simulink model "bh_4bar_model_DYN"  (R2022b)
settings: Solver=ode45  StartTime=0.0  StopTime=10  FixedStep=0.001  MaxStep=0.1  RelTol=1e-9  AbsTol=1e-9  EnableMultiTasking=on
values from neighbouring files (symbols this model uses):
  L1 = 0.4    [bh_4bar_kin_z_analysis_CLS.m]
  L2 = 1.4    [bh_4bar_kin_z_analysis_CLS.m]
  L3 = 1.2    [bh_4bar_kin_z_analysis_CLS.m]
  L4 = 1    [bh_4bar_kin_z_analysis_CLS.m]
  N = length(THE_DEG_ANG_VEC)    [bh_4bar_kin_z_analysis_CLS.m]
  X = my_stuff_T.theta_deg_vec    [bh_4bar_kin_z_analysis_CLS.m]
undefined symbols (not defined in the file or in its folder): alpha_0_rad, alpha_dot_0_rad, alpha_rad, g, H, I_G1, I_G2, I_G3, m1, m2, m3, phi_0_rad, phi_dot_0_rad, phi_rad, theta_0_rad, theta_dot_0_rad, W, Y, Z
libraries: nesl_utility x20, sm_lib x15, simulink_extras x14, bh_4bar_SL_LIB x13
(part 1 of 3)
settings Model: Creator=bhorton  LastModifiedBy=bhorton
settings SolverCC: ZeroCrossAlgorithm=Adaptive  AlgebraicLoopSolver=TrustRegion
settings DataIOCC: LimitDataPoints=on  ReturnWorkspaceOutputs=off
settings OptimizationCC: LifeSpan=inf
settings DebuggingCC: UnconnectedInputMsg=warning  UnconnectedOutputMsg=warning  UnconnectedLineMsg=warning  AllowSymbolicDim=off  PregeneratedLibrarySubsystemCodeDiagnostic=none  SFUnexpectedBacktrackingDiag=warning  SFNoUnconditionalDefaultTransitionDiag=warning  SFExecutionAtInitializationDiag=none  SFMachineParentedDataDiag=warning  ArithmeticOperatorsInVariantConditions=warning
settings ModelReferenceCC: EnableRefExpFcnMdlSchedulingChecks=on
settings SFSimCC: SimUseLocalCustomCode=off  CustomCodeUndefinedFunction=UseInterfaceOnly
settings RTWCC: RTWUseLocalCustomCode=off  DLArmComputeVersion=19.05
settings CodeAppCC: StateflowObjectComments=on
settings GRTTargetCC: TargetLangStandard=C89/C90 (ANSI)
settings ConfigComp: CovMetricSettings=dw  CovSaveCumulativeToWorkspaceVar=on  CovSaveSingleToWorkspaceVar=on  CovExternalEMLEnable=off  CovSFcnEnable=off
settings SimscapeCC: SimscapeNominalValues="[{\"value\":\"10\",\"unit\":\"V\"},{\"value\":\"1\",\"unit\":\"A\"},{\"value\":\"10\",\"unit\":\"N*m\"},{\"value\":\"10\",\"unit\":\"bar\"},{\"value\":\"100\",\"unit\":\"kJ/kg\"},{\"value\":\"1\",\"unit\":\"kW\"},{\"value\":\"300\",\"unit\":\"K\"},{\"value\":\"100\",\"unit\":\"cm^3/s\"},{\"value\":\"1\",\"unit\":\"kN\"},{\"value\":\"1\",\"unit\":\"g/cm^3\"},{\"value\":\"1\",\"unit\":\"l\"},{\"value\":\"1\",\"unit\":\"cm^2\"},{\"value\":\"60\",\"unit\":\"Hz\"}]"  SimscapeLogType=all  SimscapeLogDataHistory=10000
settings ConfigurationSet: Description=SimMechanics 2G
settings ExplorerConfigSet: InternalSimMechanicsExplorerSettings="<ExplorerConfiguration><canonicalview>default</canonicalview><AnimationSetting><BasePlaybackSpeed>1.0</BasePlaybackSpeed><PlaybackSpeedFactor>1.0</PlaybackSpeedFactor></AnimationSetting><TilePanel><TileInfo><Tiles Columns=\"1\" Count=\"1\" Rows=\"1\"><Column Weight=\"1\"/><Row Weight=\"1\"/><Tile Height=\"1\" Width=\"1\" X=\"0\" Y=\"0\"/></Tiles></TileInfo><SceneInfo><SceneViewer><BGColor><R>0.60000002384185791</R><G>0.60000002384185791</G><B>0.60000002384185791</B></BGColor><Camera><DoPerspective>off</DoPerspective><Position><X>0.674057005362880823</X><Y>0.451513124756151407</Y><Z>1.11774542835223722</Z></Position><Center><X>0.674057005362880823</X><Y>0.451513124756151407</Y><Z>-0.00200006458294343936</Z></Center><Up><X>0</X><Y>1</Y><Z>-0</Z></Up><ViewLimDist>1</ViewLimDist><YLim>0.872355052534568132</YLim><XLim>1.30853257880185225</XLim></Camera></SceneViewer></SceneInfo></TilePanel><MechEditorPanel><Cameras/><GfxPanelCameraMap/><VideoCreator><PlaybackSpeedRatio>1.0</PlaybackSpeedRatio><FrameRate>30</FrameRate><VideoFormat>Motion JPEG AVI</VideoFormat><FrameSize>auto</FrameSize></VideoCreator></MechEditorPanel></ExplorerConfiguration>"

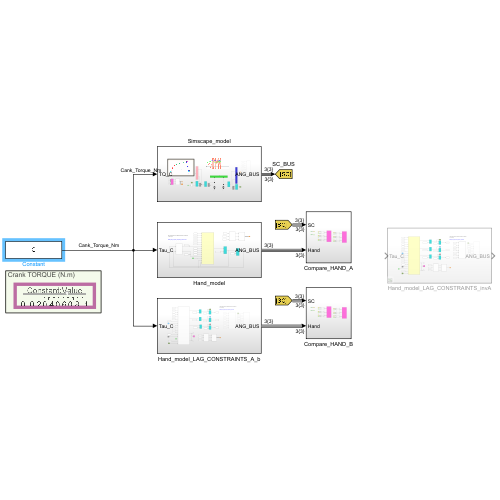
[thumbnail: Simulink's stored preview of the top-level diagram]
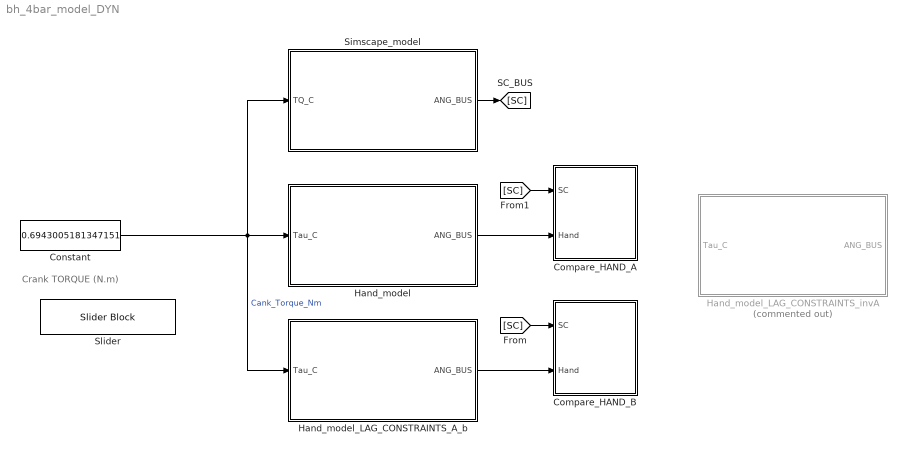
== system bh_4bar_model_DYN ==
  note: Crank TORQUE (N.m)
  Compare_HAND_A : Subsystem
  Compare_HAND_B : Subsystem
  Constant : Constant  Value=0.6943005181347151
  Hand_model : Subsystem
  Hand_model_LAG_CONSTRAINTS_A_b : Subsystem
  Hand_model_LAG_CONSTRAINTS_invA : Subsystem  Commented=on
  Simscape_model : Subsystem
  Slider : SliderBlock  ScaleMax=1
  wires:
  Constant/1 -> Hand_model_LAG_CONSTRAINTS_A_b/1(Tau_C), Simscape_model/1(TQ_C), Hand_model/1(Tau_C)  "Cank_Torque_Nm"
  Simscape_model/1(ANG_BUS) -> [SC]
  Hand_model/1(ANG_BUS) -> Compare_HAND_A/2(Hand)
  Hand_model_LAG_CONSTRAINTS_A_b/1(ANG_BUS) -> Compare_HAND_B/2(Hand)
  [SC] -> Compare_HAND_B/1(SC)
  [SC] -> Compare_HAND_A/1(SC)

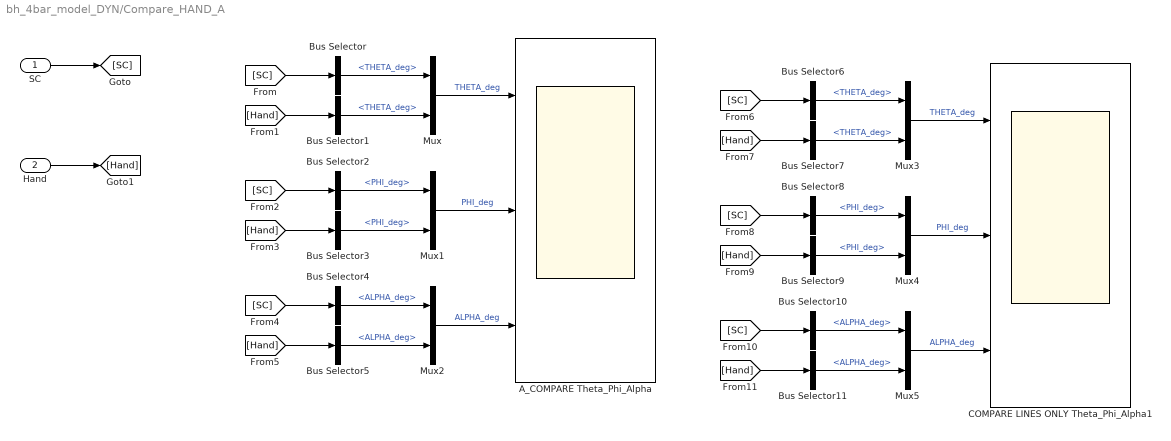
== system bh_4bar_model_DYN/Compare_HAND_A ==
  SC : Inport
  Hand : Inport  Port=2
  A_COMPARE Theta_Phi_Alpha : Scope  NumInputPorts=3
  Bus Selector{,1,6..7} (4 alike) : BusSelector  OutputSignals=THETA_deg
  Bus Selector{4..5,10..11} (4 alike) : BusSelector  OutputSignals=ALPHA_deg
  Bus Selector{2..3,8..9} (4 alike) : BusSelector  OutputSignals=PHI_deg
  COMPARE LINES ONLY Theta_Phi_Alpha1 : Scope  NumInputPorts=3
  Mux{,1..5} (6 alike) : Mux  Inputs=2
  wires:
  Hand/1 -> [Hand]
  SC/1 -> [SC]
  Mux/1 -> A_COMPARE Theta_Phi_Alpha/1  "THETA_deg"
  [SC] -> Bus Selector/1
  Bus Selector/1 -> Mux/1  "<THETA_deg>"
  [Hand] -> Bus Selector1/1
  Bus Selector1/1 -> Mux/2  "<THETA_deg>"
  Mux1/1 -> A_COMPARE Theta_Phi_Alpha/2  "PHI_deg"
  [SC] -> Bus Selector2/1
  Bus Selector3/1 -> Mux1/2  "<PHI_deg>"
  [Hand] -> Bus Selector3/1
  Bus Selector2/1 -> Mux1/1  "<PHI_deg>"
  Mux2/1 -> A_COMPARE Theta_Phi_Alpha/3  "ALPHA_deg"
  [Hand] -> Bus Selector5/1
  [SC] -> Bus Selector4/1
  Bus Selector5/1 -> Mux2/2  "<ALPHA_deg>"
  Bus Selector4/1 -> Mux2/1  "<ALPHA_deg>"
  Bus Selector10/1 -> Mux5/1  "<ALPHA_deg>"
  [Hand] -> Bus Selector11/1
  Mux5/1 -> COMPARE LINES ONLY Theta_Phi_Alpha1/3  "ALPHA_deg"
  Bus Selector11/1 -> Mux5/2  "<ALPHA_deg>"
  Mux4/1 -> COMPARE LINES ONLY Theta_Phi_Alpha1/2  "PHI_deg"
  [Hand] -> Bus Selector7/1
  Bus Selector8/1 -> Mux4/1  "<PHI_deg>"
  [SC] -> Bus Selector6/1
  Mux3/1 -> COMPARE LINES ONLY Theta_Phi_Alpha1/1  "THETA_deg"
  Bus Selector6/1 -> Mux3/1  "<THETA_deg>"
  [Hand] -> Bus Selector9/1
  [SC] -> Bus Selector8/1
  Bus Selector7/1 -> Mux3/2  "<THETA_deg>"
  [SC] -> Bus Selector10/1
  Bus Selector9/1 -> Mux4/2  "<PHI_deg>"

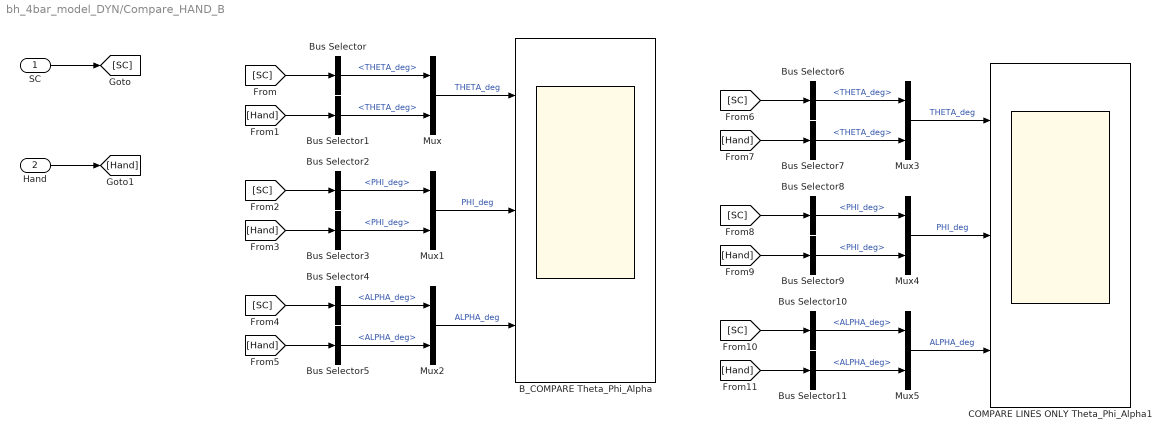
== system bh_4bar_model_DYN/Compare_HAND_B ==
  SC : Inport
  Hand : Inport  Port=2
  B_COMPARE Theta_Phi_Alpha : Scope  NumInputPorts=3
  Bus Selector{,1,6..7} (4 alike) : BusSelector  OutputSignals=THETA_deg
  Bus Selector{4..5,10..11} (4 alike) : BusSelector  OutputSignals=ALPHA_deg
  Bus Selector{2..3,8..9} (4 alike) : BusSelector  OutputSignals=PHI_deg
  COMPARE LINES ONLY Theta_Phi_Alpha1 : Scope  NumInputPorts=3
  Mux{,1..5} (6 alike) : Mux  Inputs=2
  wires:
  Hand/1 -> [Hand]
  SC/1 -> [SC]
  Mux/1 -> B_COMPARE Theta_Phi_Alpha/1  "THETA_deg"
  [SC] -> Bus Selector/1
  Bus Selector/1 -> Mux/1  "<THETA_deg>"
  [Hand] -> Bus Selector1/1
  Bus Selector1/1 -> Mux/2  "<THETA_deg>"
  Mux1/1 -> B_COMPARE Theta_Phi_Alpha/2  "PHI_deg"
  [SC] -> Bus Selector2/1
  Bus Selector3/1 -> Mux1/2  "<PHI_deg>"
  [Hand] -> Bus Selector3/1
  Bus Selector2/1 -> Mux1/1  "<PHI_deg>"
  Mux2/1 -> B_COMPARE Theta_Phi_Alpha/3  "ALPHA_deg"
  [Hand] -> Bus Selector5/1
  [SC] -> Bus Selector4/1
  Bus Selector5/1 -> Mux2/2  "<ALPHA_deg>"
  Bus Selector4/1 -> Mux2/1  "<ALPHA_deg>"
  Bus Selector10/1 -> Mux5/1  "<ALPHA_deg>"
  [Hand] -> Bus Selector11/1
  Mux5/1 -> COMPARE LINES ONLY Theta_Phi_Alpha1/3  "ALPHA_deg"
  Bus Selector11/1 -> Mux5/2  "<ALPHA_deg>"
  Mux4/1 -> COMPARE LINES ONLY Theta_Phi_Alpha1/2  "PHI_deg"
  [Hand] -> Bus Selector7/1
  Bus Selector8/1 -> Mux4/1  "<PHI_deg>"
  [SC] -> Bus Selector6/1
  Mux3/1 -> COMPARE LINES ONLY Theta_Phi_Alpha1/1  "THETA_deg"
  Bus Selector6/1 -> Mux3/1  "<THETA_deg>"
  [Hand] -> Bus Selector9/1
  [SC] -> Bus Selector8/1
  Bus Selector7/1 -> Mux3/2  "<THETA_deg>"
  [SC] -> Bus Selector10/1
  Bus Selector9/1 -> Mux4/2  "<PHI_deg>"

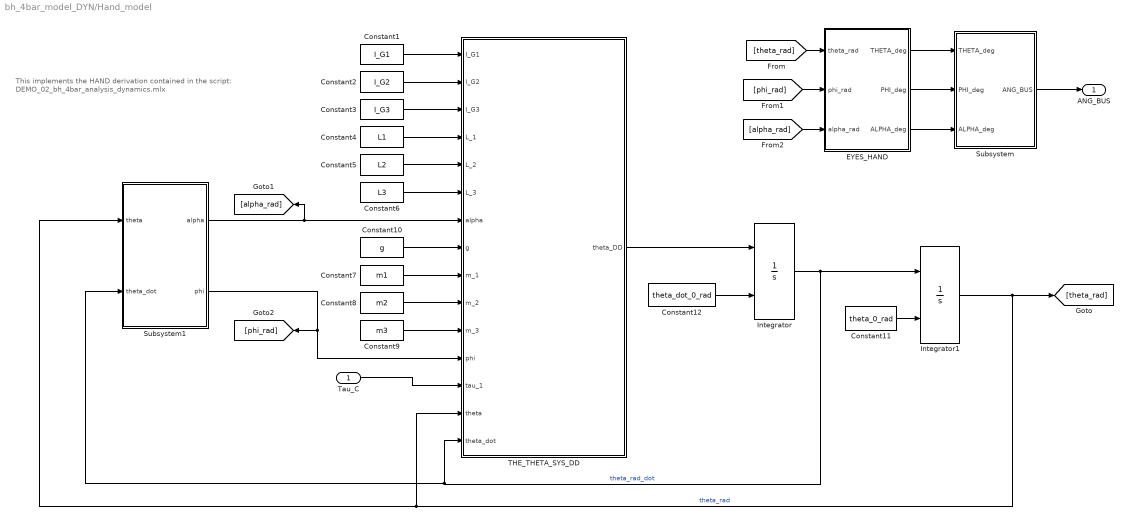
== system bh_4bar_model_DYN/Hand_model ==
  note: This implements the HAND derivation contained
      | in the script:
      |
      | DEMO_02_bh_4bar_analysis_dynamics.mlx
  Tau_C : Inport
  Constant1 : Constant  Value=I_G1
  Constant10 : Constant  Value=g
  Constant11 : Constant  Value=theta_0_rad
  Constant12 : Constant  Value=theta_dot_0_rad
  Constant2 : Constant  Value=I_G2
  Constant3 : Constant  Value=I_G3
  Constant4 : Constant  Value=L1
  Constant5 : Constant  Value=L2
  Constant6 : Constant  Value=L3
  Constant7 : Constant  Value=m1
  Constant8 : Constant  Value=m2
  Constant9 : Constant  Value=m3
  EYES_HAND : Subsystem
  Integrator : Integrator  InitialConditionSource=external
  Integrator1 : Integrator  InitialConditionSource=external
  Subsystem : Subsystem
  Subsystem1 : Subsystem
  THE_THETA_SYS_DD : MATLAB Function  TreatAsAtomicUnit=on
  ANG_BUS : Outport  VectorParamsAs1DForOutWhenUnconnected=off
  wires:
  Constant7/1 -> THE_THETA_SYS_DD/9(m_1)
  Constant8/1 -> THE_THETA_SYS_DD/10(m_2)
  Integrator/1 -> THE_THETA_SYS_DD/15(theta_dot), Subsystem1/2(theta_dot), Integrator1/1  "theta_rad_dot"
  Subsystem1/1(alpha) -> THE_THETA_SYS_DD/7(alpha), [alpha_rad]
  Constant6/1 -> THE_THETA_SYS_DD/6(L_3)
  Integrator1/1 -> [theta_rad], THE_THETA_SYS_DD/14(theta), Subsystem1/1(theta)  "theta_rad"
  Subsystem/1(ANG_BUS) -> ANG_BUS/1
  Constant5/1 -> THE_THETA_SYS_DD/5(L_2)
  EYES_HAND/2(PHI_deg) -> Subsystem/2(PHI_deg)
  EYES_HAND/1(THETA_deg) -> Subsystem/1(THETA_deg)
  EYES_HAND/3(ALPHA_deg) -> Subsystem/3(ALPHA_deg)
  Subsystem1/2(phi) -> THE_THETA_SYS_DD/12(phi), [phi_rad]
  [theta_rad] -> EYES_HAND/1(theta_rad)
  [phi_rad] -> EYES_HAND/2(phi_rad)
  THE_THETA_SYS_DD/1(theta_DD) -> Integrator/1
  [alpha_rad] -> EYES_HAND/3(alpha_rad)
  Constant3/1 -> THE_THETA_SYS_DD/3(I_G3)
  Constant2/1 -> THE_THETA_SYS_DD/2(I_G2)
  Constant4/1 -> THE_THETA_SYS_DD/4(L_1)
  Constant10/1 -> THE_THETA_SYS_DD/8(g)
  Constant9/1 -> THE_THETA_SYS_DD/11(m_3)
  Constant1/1 -> THE_THETA_SYS_DD/1(I_G1)
  Tau_C/1 -> THE_THETA_SYS_DD/13(tau_1)
  Constant12/1 -> Integrator/2
  Constant11/1 -> Integrator1/2

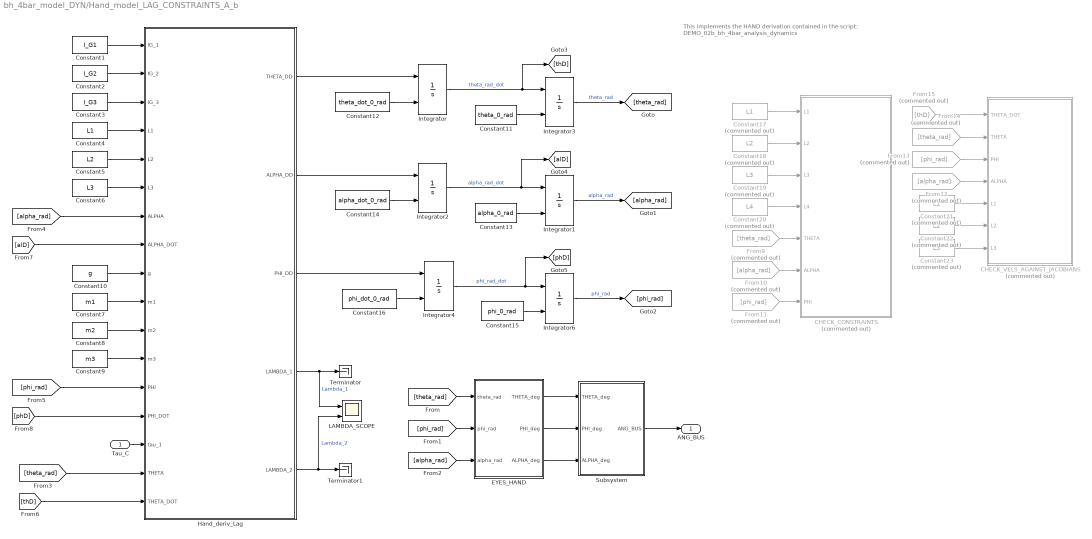
== system bh_4bar_model_DYN/Hand_model_LAG_CONSTRAINTS_A_b ==
  note: This implements the HAND derivation contained
      | in the script:
      |
      | DEMO_02b_bh_4bar_analysis_dynamics
  Tau_C : Inport
  CHECK_CONSTRAINTS : Subsystem  Commented=on
  CHECK_VELS_AGAINST_JACOBIANS : Subsystem  Commented=on
  Constant1 : Constant  Value=I_G1
  Constant10 : Constant  Value=g
  Constant11 : Constant  Value=theta_0_rad
  Constant12 : Constant  Value=theta_dot_0_rad
  Constant13 : Constant  Value=alpha_0_rad
  Constant14 : Constant  Value=alpha_dot_0_rad
  Constant15 : Constant  Value=phi_0_rad
  Constant16 : Constant  Value=phi_dot_0_rad
  Constant17 : Constant  Commented=on  Value=L1
  Constant18 : Constant  Commented=on  Value=L2
  Constant19 : Constant  Commented=on  Value=L3
  Constant2 : Constant  Value=I_G2
  Constant20 : Constant  Commented=on  Value=L4
  Constant21 : Constant  Commented=on  Value=L1
  Constant22 : Constant  Commented=on  Value=L2
  Constant23 : Constant  Commented=on  Value=L3
  Constant3 : Constant  Value=I_G3
  Constant4 : Constant  Value=L1
  Constant5 : Constant  Value=L2
  Constant6 : Constant  Value=L3
  Constant7 : Constant  Value=m1
  Constant8 : Constant  Value=m2
  Constant9 : Constant  Value=m3
  EYES_HAND : Subsystem
  From10 : From  Commented=on  GotoTag=alpha_rad
  From11 : From  Commented=on  GotoTag=phi_rad
  From12 : From  Commented=on  GotoTag=alpha_rad
  From13 : From  Commented=on  GotoTag=phi_rad
  From14 : From  Commented=on  GotoTag=theta_rad
  From15 : From  Commented=on  GotoTag=thD
  From9 : From  Commented=on  GotoTag=theta_rad
  Hand_deriv_Lag : Subsystem
  Integrator : Integrator  InitialConditionSource=external
  Integrator1 : Integrator  InitialConditionSource=external  WrapState=on
  Integrator2 : Integrator  InitialConditionSource=external
  Integrator3 : Integrator  InitialConditionSource=external  WrapState=on
  Integrator4 : Integrator  InitialConditionSource=external
  Integrator6 : Integrator  InitialConditionSource=external  WrapState=on
  LAMBDA_SCOPE : Scope  NumInputPorts=2
  Subsystem : Subsystem
  Terminator : Terminator
  Terminator1 : Terminator
  ANG_BUS : Outport  VectorParamsAs1DForOutWhenUnconnected=off
  wires:
  Constant7/1 -> Hand_deriv_Lag/10(m1)
  Constant8/1 -> Hand_deriv_Lag/11(m2)
  Integrator/1 -> Integrator3/1, [thD]  "theta_rad_dot"
  Constant6/1 -> Hand_deriv_Lag/6(L3)
  Integrator3/1 -> [theta_rad]  "theta_rad"
  Subsystem/1(ANG_BUS) -> ANG_BUS/1
  Constant5/1 -> Hand_deriv_Lag/5(L2)
  EYES_HAND/2(PHI_deg) -> Subsystem/2(PHI_deg)
  EYES_HAND/1(THETA_deg) -> Subsystem/1(THETA_deg)
  EYES_HAND/3(ALPHA_deg) -> Subsystem/3(ALPHA_deg)
  [theta_rad] -> EYES_HAND/1(theta_rad)
  [phi_rad] -> EYES_HAND/2(phi_rad)
  Hand_deriv_Lag/1(THETA_DD) -> Integrator/1
  [alpha_rad] -> EYES_HAND/3(alpha_rad)
  Constant3/1 -> Hand_deriv_Lag/3(IG_3)
  Constant2/1 -> Hand_deriv_Lag/2(IG_2)
  Constant4/1 -> Hand_deriv_Lag/4(L1)
  Constant10/1 -> Hand_deriv_Lag/9(g)
  Constant9/1 -> Hand_deriv_Lag/12(m3)
  Constant1/1 -> Hand_deriv_Lag/1(IG_1)
  Tau_C/1 -> Hand_deriv_Lag/15(tau_1)
  Constant12/1 -> Integrator/2
  Constant11/1 -> Integrator3/2
  Integrator2/1 -> Integrator1/1, [alD]  "alpha_rad_dot"
  Hand_deriv_Lag/2(ALPHA_DD) -> Integrator2/1
  Constant13/1 -> Integrator1/2
  Integrator1/1 -> [alpha_rad]  "alpha_rad"
  Constant14/1 -> Integrator2/2
  Constant15/1 -> Integrator6/2
  Integrator4/1 -> Integrator6/1, [phD]  "phi_rad_dot"
  Integrator6/1 -> [phi_rad]  "phi_rad"
  Constant16/1 -> Integrator4/2
  Hand_deriv_Lag/3(PHI_DD) -> Integrator4/1
  Hand_deriv_Lag/4(LAMBDA_1) -> LAMBDA_SCOPE/1, Terminator/1  "Lambda_1"
  Hand_deriv_Lag/5(LAMBDA_2) -> LAMBDA_SCOPE/2, Terminator1/1  "Lambda_2"
  [theta_rad] -> Hand_deriv_Lag/16(THETA)
  [thD] -> Hand_deriv_Lag/17(THETA_DOT)
  [phD] -> Hand_deriv_Lag/14(PHI_DOT)
  [phi_rad] -> Hand_deriv_Lag/13(PHI)
  [alD] -> Hand_deriv_Lag/8(ALPHA_DOT)
  [alpha_rad] -> Hand_deriv_Lag/7(ALPHA)
  Constant17/1 -> CHECK_CONSTRAINTS/1(L1)
  Constant18/1 -> CHECK_CONSTRAINTS/2(L2)
  Constant19/1 -> CHECK_CONSTRAINTS/3(L3)
  Constant20/1 -> CHECK_CONSTRAINTS/4(L4)
  From9/1 -> CHECK_CONSTRAINTS/5(THETA)
  From10/1 -> CHECK_CONSTRAINTS/6(ALPHA)
  From11/1 -> CHECK_CONSTRAINTS/7(PHI)
  From15/1 -> CHECK_VELS_AGAINST_JACOBIANS/1(THETA_DOT)
  From14/1 -> CHECK_VELS_AGAINST_JACOBIANS/2(THETA)
  From13/1 -> CHECK_VELS_AGAINST_JACOBIANS/3(PHI)
  From12/1 -> CHECK_VELS_AGAINST_JACOBIANS/4(ALPHA)
  Constant21/1 -> CHECK_VELS_AGAINST_JACOBIANS/5(L1)
  Constant22/1 -> CHECK_VELS_AGAINST_JACOBIANS/6(L2)
  Constant23/1 -> CHECK_VELS_AGAINST_JACOBIANS/7(L3)

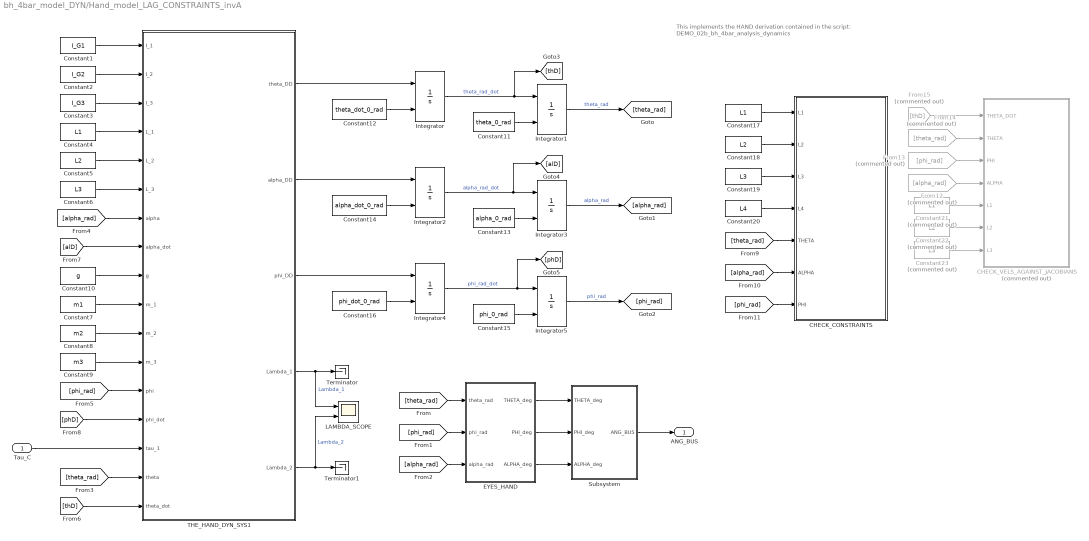
== system bh_4bar_model_DYN/Hand_model_LAG_CONSTRAINTS_invA ==
  note: This implements the HAND derivation contained
      | in the script:
      |
      | DEMO_02b_bh_4bar_analysis_dynamics
  Tau_C : Inport
  CHECK_CONSTRAINTS : Subsystem
  CHECK_VELS_AGAINST_JACOBIANS : Subsystem  Commented=on
  Constant1 : Constant  Value=I_G1
  Constant10 : Constant  Value=g
  Constant11 : Constant  Value=theta_0_rad
  Constant12 : Constant  Value=theta_dot_0_rad
  Constant13 : Constant  Value=alpha_0_rad
  Constant14 : Constant  Value=alpha_dot_0_rad
  Constant15 : Constant  Value=phi_0_rad
  Constant16 : Constant  Value=phi_dot_0_rad
  Constant17 : Constant  Value=L1
  Constant18 : Constant  Value=L2
  Constant19 : Constant  Value=L3
  Constant2 : Constant  Value=I_G2
  Constant20 : Constant  Value=L4
  Constant21 : Constant  Commented=on  Value=L1
  Constant22 : Constant  Commented=on  Value=L2
  Constant23 : Constant  Commented=on  Value=L3
  Constant3 : Constant  Value=I_G3
  Constant4 : Constant  Value=L1
  Constant5 : Constant  Value=L2
  Constant6 : Constant  Value=L3
  Constant7 : Constant  Value=m1
  Constant8 : Constant  Value=m2
  Constant9 : Constant  Value=m3
  EYES_HAND : Subsystem
  From12 : From  Commented=on  GotoTag=alpha_rad
  From13 : From  Commented=on  GotoTag=phi_rad
  From14 : From  Commented=on  GotoTag=theta_rad
  From15 : From  Commented=on  GotoTag=thD
  Integrator : Integrator  InitialConditionSource=external
  Integrator1 : Integrator  InitialConditionSource=external  WrapState=on
  Integrator2 : Integrator  InitialConditionSource=external
  Integrator3 : Integrator  InitialConditionSource=external  WrapState=on
  Integrator4 : Integrator  InitialConditionSource=external
  Integrator5 : Integrator  InitialConditionSource=external  WrapState=on
  LAMBDA_SCOPE : Scope  NumInputPorts=2
  Subsystem : Subsystem
  THE_HAND_DYN_SYS1 : MATLAB Function  TreatAsAtomicUnit=on
  Terminator : Terminator
  Terminator1 : Terminator
  ANG_BUS : Outport  VectorParamsAs1DForOutWhenUnconnected=off
  wires:
  Constant7/1 -> THE_HAND_DYN_SYS1/10(m_1)
  Constant8/1 -> THE_HAND_DYN_SYS1/11(m_2)
  Integrator/1 -> [thD], Integrator1/1  "theta_rad_dot"
  Constant6/1 -> THE_HAND_DYN_SYS1/6(L_3)
  Integrator1/1 -> [theta_rad]  "theta_rad"
  Subsystem/1(ANG_BUS) -> ANG_BUS/1
  Constant5/1 -> THE_HAND_DYN_SYS1/5(L_2)
  EYES_HAND/2(PHI_deg) -> Subsystem/2(PHI_deg)
  EYES_HAND/1(THETA_deg) -> Subsystem/1(THETA_deg)
  EYES_HAND/3(ALPHA_deg) -> Subsystem/3(ALPHA_deg)
  [theta_rad] -> EYES_HAND/1(theta_rad)
  [phi_rad] -> EYES_HAND/2(phi_rad)
  THE_HAND_DYN_SYS1/1(theta_DD) -> Integrator/1
  [alpha_rad] -> EYES_HAND/3(alpha_rad)
  Constant3/1 -> THE_HAND_DYN_SYS1/3(I_3)
  Constant2/1 -> THE_HAND_DYN_SYS1/2(I_2)
  Constant4/1 -> THE_HAND_DYN_SYS1/4(L_1)
  Constant10/1 -> THE_HAND_DYN_SYS1/9(g)
  Constant9/1 -> THE_HAND_DYN_SYS1/12(m_3)
  Constant1/1 -> THE_HAND_DYN_SYS1/1(I_1)
  Tau_C/1 -> THE_HAND_DYN_SYS1/15(tau_1)
  Constant12/1 -> Integrator/2
  Constant11/1 -> Integrator1/2
  Integrator2/1 -> [alD], Integrator3/1  "alpha_rad_dot"
  THE_HAND_DYN_SYS1/2(alpha_DD) -> Integrator2/1
  Constant13/1 -> Integrator3/2
  Integrator3/1 -> [alpha_rad]  "alpha_rad"
  Constant14/1 -> Integrator2/2
  Constant15/1 -> Integrator5/2
  Integrator4/1 -> [phD], Integrator5/1  "phi_rad_dot"
  Integrator5/1 -> [phi_rad]  "phi_rad"
  Constant16/1 -> Integrator4/2
  THE_HAND_DYN_SYS1/3(phi_DD) -> Integrator4/1
  THE_HAND_DYN_SYS1/4(Lambda_1) -> LAMBDA_SCOPE/1, Terminator/1  "Lambda_1"
  THE_HAND_DYN_SYS1/5(Lambda_2) -> LAMBDA_SCOPE/2, Terminator1/1  "Lambda_2"
  [theta_rad] -> THE_HAND_DYN_SYS1/16(theta)
  [thD] -> THE_HAND_DYN_SYS1/17(theta_dot)
  [phD] -> THE_HAND_DYN_SYS1/14(phi_dot)
  [phi_rad] -> THE_HAND_DYN_SYS1/13(phi)
  [alD] -> THE_HAND_DYN_SYS1/8(alpha_dot)
  [alpha_rad] -> THE_HAND_DYN_SYS1/7(alpha)
  Constant17/1 -> CHECK_CONSTRAINTS/1(L1)
  Constant18/1 -> CHECK_CONSTRAINTS/2(L2)
  Constant19/1 -> CHECK_CONSTRAINTS/3(L3)
  Constant20/1 -> CHECK_CONSTRAINTS/4(L4)
  [theta_rad] -> CHECK_CONSTRAINTS/5(THETA)
  [alpha_rad] -> CHECK_CONSTRAINTS/6(ALPHA)
  [phi_rad] -> CHECK_CONSTRAINTS/7(PHI)
  From15/1 -> CHECK_VELS_AGAINST_JACOBIANS/1(THETA_DOT)
  From14/1 -> CHECK_VELS_AGAINST_JACOBIANS/2(THETA)
  From13/1 -> CHECK_VELS_AGAINST_JACOBIANS/3(PHI)
  From12/1 -> CHECK_VELS_AGAINST_JACOBIANS/4(ALPHA)
  Constant21/1 -> CHECK_VELS_AGAINST_JACOBIANS/5(L1)
  Constant22/1 -> CHECK_VELS_AGAINST_JACOBIANS/6(L2)
  Constant23/1 -> CHECK_VELS_AGAINST_JACOBIANS/7(L3)

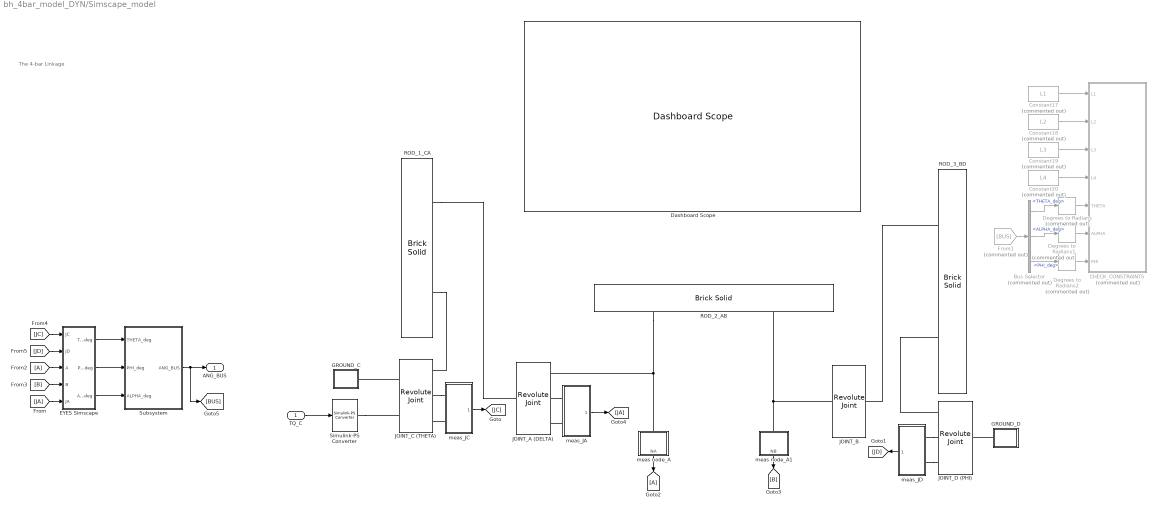
== system bh_4bar_model_DYN/Simscape_model ==
  note: The 4-bar Linkage
  TQ_C : Inport
  Bus Selector : BusSelector  Commented=on  OutputSignals=THETA_deg,ALPHA_deg,PHI_deg
  CHECK_CONSTRAINTS : Subsystem  Commented=on
  Constant17 : Constant  Commented=on  Value=L1
  Constant18 : Constant  Commented=on  Value=L2
  Constant19 : Constant  Commented=on  Value=L3
  Constant20 : Constant  Commented=on  Value=L4
  Dashboard Scope : DashboardScope
  Degrees to Radians : simulink_extras/Transformations/Degrees to Radians  Commented=on
  Degrees to Radians1 : simulink_extras/Transformations/Degrees to Radians  Commented=on
  Degrees to Radians2 : simulink_extras/Transformations/Degrees to Radians  Commented=on
  EYES Simscape : Subsystem
  From1 : From  Commented=on  GotoTag=BUS
  From2 : From
  GROUND_C : Subsystem
  GROUND_D : Subsystem
  Goto2 : Goto
  JOINT_A (DELTA) : sm_lib/Joints/Revolute Joint  JointMode=Normal  SenseConstraintForce=off  SenseConstraintForceX=off  SenseConstraintForceY=off  SenseConstraintForceZ=off  SenseConstraintTorque=off  SenseConstraintTorqueX=off  SenseConstraintTorqueY=off  SenseConstraintTorqueZ=off  SenseTotalForce=off  SenseTotalForceX=off  SenseTotalForceY=off  SenseTotalForceZ=off  SenseTotalTorque=off  SenseTotalTorqueX=off  SenseTotalTorqueY=off  SenseTotalTorqueZ=off  CompositeWrenchDir=FollowerOnBase  CompositeWrenchFrame=BaseFrame  EquilibriumPosition=0  EquilibriumPositionUnits=deg  SpringStiffness=0  SpringStiffnessUnits=N*m/deg  DampingCoefficient=0  DampingCoefficientUnits=N*m/(deg/s)  TorqueActuationMode=NoTorque  MotionActuationMode=ComputedMotion  SensePosition=on  SenseVelocity=on  SenseAcceleration=off  SenseTorqueForce=off  SenseLowerLimitTorqueForce=off  SenseUpperLimitTorqueForce=off  LowerLimitSpecify=off  LowerLimitBound=-90  LowerLimitBoundUnits=deg  LowerLimitStiffness=1e4  LowerLimitStiffnessUnits=N*m/deg  LowerLimitDamping=10  LowerLimitDampingUnits=N*m/(deg/s)  LowerLimitTransitionRegionWidth=0.1  LowerLimitTransitionRegionWidthUnits=deg  UpperLimitSpecify=off  UpperLimitBound=90  UpperLimitBoundUnits=deg  UpperLimitStiffness=1e4  UpperLimitStiffnessUnits=N*m/deg  UpperLimitDamping=10  UpperLimitDampingUnits=N*m/(deg/s)  UpperLimitTransitionRegionWidth=0.1  UpperLimitTransitionRegionWidthUnits=deg  PositionTargetSpecify=off  PositionTargetPriority=High  PositionTargetValue=0  PositionTargetValueUnits=deg  VelocityTargetSpecify=off  VelocityTargetPriority=High  VelocityTargetValue=0  VelocityTargetValueUnits=deg/s
  JOINT_B : sm_lib/Joints/Revolute Joint  JointMode=Normal  SenseConstraintForce=off  SenseConstraintForceX=off  SenseConstraintForceY=off  SenseConstraintForceZ=off  SenseConstraintTorque=off  SenseConstraintTorqueX=off  SenseConstraintTorqueY=off  SenseConstraintTorqueZ=off  SenseTotalForce=off  SenseTotalForceX=off  SenseTotalForceY=off  SenseTotalForceZ=off  SenseTotalTorque=off  SenseTotalTorqueX=off  SenseTotalTorqueY=off  SenseTotalTorqueZ=off  CompositeWrenchDir=FollowerOnBase  CompositeWrenchFrame=BaseFrame  EquilibriumPosition=0  EquilibriumPositionUnits=deg  SpringStiffness=0  SpringStiffnessUnits=N*m/deg  DampingCoefficient=0  DampingCoefficientUnits=N*m/(deg/s)  TorqueActuationMode=NoTorque  MotionActuationMode=ComputedMotion  SensePosition=off  SenseVelocity=off  SenseAcceleration=off  SenseTorqueForce=off  SenseLowerLimitTorqueForce=off  SenseUpperLimitTorqueForce=off  LowerLimitSpecify=off  LowerLimitBound=-90  LowerLimitBoundUnits=deg  LowerLimitStiffness=1e4  LowerLimitStiffnessUnits=N*m/deg  LowerLimitDamping=10  LowerLimitDampingUnits=N*m/(deg/s)  LowerLimitTransitionRegionWidth=0.1  LowerLimitTransitionRegionWidthUnits=deg  UpperLimitSpecify=off  UpperLimitBound=90  UpperLimitBoundUnits=deg  UpperLimitStiffness=1e4  UpperLimitStiffnessUnits=N*m/deg  UpperLimitDamping=10  UpperLimitDampingUnits=N*m/(deg/s)  UpperLimitTransitionRegionWidth=0.1  UpperLimitTransitionRegionWidthUnits=deg  PositionTargetSpecify=off  PositionTargetPriority=High  PositionTargetValue=0  PositionTargetValueUnits=deg  VelocityTargetSpecify=off  VelocityTargetPriority=High  VelocityTargetValue=0  VelocityTargetValueUnits=deg/s
  JOINT_C (THETA) : sm_lib/Joints/Revolute Joint  JointMode=Normal  SenseConstraintForce=off  SenseConstraintForceX=off  SenseConstraintForceY=off  SenseConstraintForceZ=off  SenseConstraintTorque=off  SenseConstraintTorqueX=off  SenseConstraintTorqueY=off  SenseConstraintTorqueZ=off  SenseTotalForce=off  SenseTotalForceX=off  SenseTotalForceY=off  SenseTotalForceZ=off  SenseTotalTorque=off  SenseTotalTorqueX=off  SenseTotalTorqueY=off  SenseTotalTorqueZ=off  CompositeWrenchDir=FollowerOnBase  CompositeWrenchFrame=BaseFrame  EquilibriumPosition=0  EquilibriumPositionUnits=deg  SpringStiffness=0  SpringStiffnessUnits=N*m/deg  DampingCoefficient=0  DampingCoefficientUnits=N*m/(deg/s)  TorqueActuationMode=InputTorque  MotionActuationMode=ComputedMotion  SensePosition=on  SenseVelocity=on  SenseAcceleration=off  SenseTorqueForce=off  SenseLowerLimitTorqueForce=off  SenseUpperLimitTorqueForce=off  LowerLimitSpecify=off  LowerLimitBound=-90  LowerLimitBoundUnits=deg  LowerLimitStiffness=1e4  LowerLimitStiffnessUnits=N*m/deg  LowerLimitDamping=10  LowerLimitDampingUnits=N*m/(deg/s)  LowerLimitTransitionRegionWidth=0.1  LowerLimitTransitionRegionWidthUnits=deg  UpperLimitSpecify=off  UpperLimitBound=90  UpperLimitBoundUnits=deg  UpperLimitStiffness=1e4  UpperLimitStiffnessUnits=N*m/deg  UpperLimitDamping=10  UpperLimitDampingUnits=N*m/(deg/s)  UpperLimitTransitionRegionWidth=0.1  UpperLimitTransitionRegionWidthUnits=deg  PositionTargetSpecify=on  PositionTargetPriority=High  PositionTargetValue=joints.C.ang_degs  PositionTargetValueUnits=deg  VelocityTargetSpecify=on  VelocityTargetPriority=High  VelocityTargetValue=joints.C.vel_degs  VelocityTargetValueUnits=deg/s
      settings: AttributesFormatString=|
      | init_pos =%<PositionTargetValue>
      | %<PositionTargetValueUnits>
      | init_VEL =
      | %<VelocityTargetValue>
      | %<VelocityTargetValueUnits>
  JOINT_D (PHI) : sm_lib/Joints/Revolute Joint  JointMode=Normal  SenseConstraintForce=off  SenseConstraintForceX=off  SenseConstraintForceY=off  SenseConstraintForceZ=off  SenseConstraintTorque=off  SenseConstraintTorqueX=off  SenseConstraintTorqueY=off  SenseConstraintTorqueZ=off  SenseTotalForce=off  SenseTotalForceX=off  SenseTotalForceY=off  SenseTotalForceZ=off  SenseTotalTorque=off  SenseTotalTorqueX=off  SenseTotalTorqueY=off  SenseTotalTorqueZ=off  CompositeWrenchDir=FollowerOnBase  CompositeWrenchFrame=BaseFrame  EquilibriumPosition=0  EquilibriumPositionUnits=deg  SpringStiffness=0  SpringStiffnessUnits=N*m/deg  DampingCoefficient=0  DampingCoefficientUnits=N*m/(deg/s)  TorqueActuationMode=NoTorque  MotionActuationMode=ComputedMotion  SensePosition=on  SenseVelocity=on  SenseAcceleration=off  SenseTorqueForce=off  SenseLowerLimitTorqueForce=off  SenseUpperLimitTorqueForce=off  LowerLimitSpecify=off  LowerLimitBound=-90  LowerLimitBoundUnits=deg  LowerLimitStiffness=1e4  LowerLimitStiffnessUnits=N*m/deg  LowerLimitDamping=10  LowerLimitDampingUnits=N*m/(deg/s)  LowerLimitTransitionRegionWidth=0.1  LowerLimitTransitionRegionWidthUnits=deg  UpperLimitSpecify=off  UpperLimitBound=90  UpperLimitBoundUnits=deg  UpperLimitStiffness=1e4  UpperLimitStiffnessUnits=N*m/deg  UpperLimitDamping=10  UpperLimitDampingUnits=N*m/(deg/s)  UpperLimitTransitionRegionWidth=0.1  UpperLimitTransitionRegionWidthUnits=deg  PositionTargetSpecify=on  PositionTargetPriority=High  PositionTargetValue=joints.D.ang_degs  PositionTargetValueUnits=deg  VelocityTargetSpecify=off  VelocityTargetPriority=High  VelocityTargetValue=0  VelocityTargetValueUnits=deg/s
      settings: AttributesFormatString=|
      | init_pos =%<PositionTargetValue>
      | %<PositionTargetValueUnits>
  ROD_1_CA : sm_lib/Body Elements/Brick Solid  GraphicAmbientColor=[0.15 0.15 0.15 1.0]  BasedOnType=Density  BrickDimensions=[L1,H,W]  BrickDimensionUnits=m  CenterOfMass=[0 0 0]  CenterOfMassUnits=m  GraphicDiffuseColor=[1.0 0.4 0.6]  Density=density  DensityUnits=kg/m^3  DoExposeReferenceFrame=on  GraphicEmissiveColor=[0.0 0.0 0.0 1.0]  ExportEntireGeometry=off  SerializedFrames=<Frames><Frame><Id>Frame2</Id><Value><Name>A</Name><Origin><Source>GeometricFeature</Source><FeatureName>+z +x curve</FeatureName></Origin><PrimaryAxis><DefinedDirection>+Z</DefinedDirection><Source>ReferenceFrame</Source><SourceDirection>+Z</SourceDirection><FeatureName></FeatureName></PrimaryAxis><SecondaryAxis><DefinedDirection>+X</DefinedDirection><Source>ReferenceFrame</Source><SourceDirection>+X</SourceDirection><FeatureName></FeatureName></SecondaryAxis></Value></Frame><Frame><Id>Frame3</Id><Value><Name>C</Name><Origin><Source>GeometricFeature</Source><FeatureName>+z -x curve</FeatureName></Origin><PrimaryAxis><DefinedDirection>+Z</DefinedDirection><Source>ReferenceFrame</Source><SourceDirection>+Z</SourceDirection><FeatureName></FeatureName></PrimaryAxis><SecondaryAxis><DefinedDirection>+X</DefinedDirection><Source>ReferenceFrame</Source><SourceDirection>+X</SourceDirection><FeatureName></FeatureName></SecondaryAxis></Value></Frame></Frames>  MarkerShape=Sphere  MarkerSize=10  GraphicType=FromGeometry  InertiaType=CalculateFromGeometry  Mass=1  MassUnits=kg  MomentsOfInertia=[1 1 1]  MomentsOfInertiaUnits=kg*m^2  GraphicOpacity=1.0  ProductsOfInertia=[0 0 0]  ProductsOfInertiaUnits=kg*m^2  GraphicShininess=75  GraphicSpecularColor=[0.5 0.5 0.5 1.0]  GraphicVisPropType=SimpleVisualProperties
  ROD_2_AB : sm_lib/Body Elements/Brick Solid  GraphicAmbientColor=[0.15 0.15 0.15 1.0]  BasedOnType=Density  BrickDimensions=[L2,H,W]  BrickDimensionUnits=m  CenterOfMass=[0 0 0]  CenterOfMassUnits=m  GraphicDiffuseColor=[0.0 1.0 0.2]  Density=density  DensityUnits=kg/m^3  DoExposeReferenceFrame=on  GraphicEmissiveColor=[0.0 0.0 0.0 1.0]  ExportEntireGeometry=off  SerializedFrames=<Frames><Frame><Id>Frame1</Id><Value><Name>A</Name><Origin><Source>GeometricFeature</Source><FeatureName>+z -x curve</FeatureName></Origin><PrimaryAxis><DefinedDirection>+Z</DefinedDirection><Source>ReferenceFrame</Source><SourceDirection>+Z</SourceDirection><FeatureName></FeatureName></PrimaryAxis><SecondaryAxis><DefinedDirection>+X</DefinedDirection><Source>ReferenceFrame</Source><SourceDirection>+X</SourceDirection><FeatureName></FeatureName></SecondaryAxis></Value></Frame><Frame><Id>Frame2</Id><Value><Name>B</Name><Origin><Source>GeometricFeature</Source><FeatureName>+z +x curve</FeatureName></Origin><PrimaryAxis><DefinedDirection>+Z</DefinedDirection><Source>ReferenceFrame</Source><SourceDirection>+Z</SourceDirection><FeatureName></FeatureName></PrimaryAxis><SecondaryAxis><DefinedDirection>+X</DefinedDirection><Source>ReferenceFrame</Source><SourceDirection>+X</SourceDirection><FeatureName></FeatureName></SecondaryAxis></Value></Frame></Frames>  MarkerShape=Sphere  MarkerSize=10  GraphicType=FromGeometry  InertiaType=CalculateFromGeometry  Mass=1  MassUnits=kg  MomentsOfInertia=[1 1 1]  MomentsOfInertiaUnits=kg*m^2  GraphicOpacity=1.0  ProductsOfInertia=[0 0 0]  ProductsOfInertiaUnits=kg*m^2  GraphicShininess=75  GraphicSpecularColor=[0.5 0.5 0.5 1.0]  GraphicVisPropType=SimpleVisualProperties
  ROD_3_BD : sm_lib/Body Elements/Brick Solid  GraphicAmbientColor=[0.15 0.15 0.15 1.0]  BasedOnType=Density  BrickDimensions=[L3,H,W]  BrickDimensionUnits=m  CenterOfMass=[0 0 0]  CenterOfMassUnits=m  GraphicDiffuseColor=[0.2 0.2 1.0]  Density=density  DensityUnits=kg/m^3  DoExposeReferenceFrame=on  GraphicEmissiveColor=[0.0 0.0 0.0 1.0]  ExportEntireGeometry=off  SerializedFrames=<Frames><Frame><Id>Frame1</Id><Value><Name>B</Name><Origin><Source>GeometricFeature</Source><FeatureName>+z +x curve</FeatureName></Origin><PrimaryAxis><DefinedDirection>+Z</DefinedDirection><Source>ReferenceFrame</Source><SourceDirection>+Z</SourceDirection><FeatureName></FeatureName></PrimaryAxis><SecondaryAxis><DefinedDirection>+X</DefinedDirection><Source>ReferenceFrame</Source><SourceDirection>+X</SourceDirection><FeatureName></FeatureName></SecondaryAxis></Value></Frame><Frame><Id>Frame2</Id><Value><Name>D</Name><Origin><Source>GeometricFeature</Source><FeatureName>+z -x curve</FeatureName></Origin><PrimaryAxis><DefinedDirection>+Z</DefinedDirection><Source>ReferenceFrame</Source><SourceDirection>+Z</SourceDirection><FeatureName></FeatureName></PrimaryAxis><SecondaryAxis><DefinedDirection>+X</DefinedDirection><Source>ReferenceFrame</Source><SourceDirection>+X</SourceDirection><FeatureName></FeatureName></SecondaryAxis></Value></Frame></Frames>  MarkerShape=Sphere  MarkerSize=10  GraphicType=FromGeometry  InertiaType=CalculateFromGeometry  Mass=1  MassUnits=kg  MomentsOfInertia=[1 1 1]  MomentsOfInertiaUnits=kg*m^2  GraphicOpacity=1.0  ProductsOfInertia=[0 0 0]  ProductsOfInertiaUnits=kg*m^2  GraphicShininess=75  GraphicSpecularColor=[0.5 0.5 0.5 1.0]  GraphicVisPropType=SimpleVisualProperties
  Simulink-PS Converter : nesl_utility/Simulink-PS Converter  PhysicalDomain=network_engine_domain  SubClassName=ps_input  LeftPortType=input  RightPortType=output  PseudoPeriodic=off  Frequencies=[]  NoiseDistribution=none  NoiseParameters=[]  Unit=N*m  AffineConversion=off  FilteringAndDerivatives=filter  SimscapeFilterOrder=1  InputFilterTimeConstant=0.001  UdotUserProvided=2
  Subsystem : Subsystem
  meas node_A : Subsystem
  meas node_A1 : Subsystem
  meas_JA : Subsystem
  meas_JC : Subsystem
  meas_JD : Subsystem
  ANG_BUS : Outport  VectorParamsAs1DForOutWhenUnconnected=off
  wires:
  [JC] -> EYES Simscape/1(JC)
  meas_JC/1(PV_BUS) -> [JC]
  [JA] -> EYES Simscape/5(JA)
  [B] -> EYES Simscape/4(B)
  EYES Simscape/3(ALPHA_deg) -> Subsystem/3(ALPHA_deg)
  TQ_C/1 -> Simulink-PS Converter/1
  [JD] -> EYES Simscape/2(JD)
  From2/1 -> EYES Simscape/3(A)
  meas_JA/1(PV_BUS) -> [JA]
  EYES Simscape/1(THETA_deg) -> Subsystem/1(THETA_deg)
  meas_JD/1(PV_BUS) -> [JD]
  EYES Simscape/2(PHI_deg) -> Subsystem/2(PHI_deg)
  Subsystem/1(ANG_BUS) -> [BUS], ANG_BUS/1
  meas node_A/1(NA) -> Goto2/1
  meas node_A1/1(NB) -> [B]
  Constant20/1 -> CHECK_CONSTRAINTS/4(L4)
  Degrees to Radians1/1 -> CHECK_CONSTRAINTS/6(ALPHA)
  Degrees to Radians/1 -> CHECK_CONSTRAINTS/5(THETA)
  Constant19/1 -> CHECK_CONSTRAINTS/3(L3)
  Constant17/1 -> CHECK_CONSTRAINTS/1(L1)
  Constant18/1 -> CHECK_CONSTRAINTS/2(L2)
  Degrees to Radians2/1 -> CHECK_CONSTRAINTS/7(PHI)
  From1/1 -> Bus Selector/1
  Bus Selector/3 -> Degrees to Radians2/1  "<PHI_deg>"
  Bus Selector/2 -> Degrees to Radians1/1  "<ALPHA_deg>"
  Bus Selector/1 -> Degrees to Radians/1  "<THETA_deg>"
  connections:
  meas_JD/LConn2 -- JOINT_D (PHI)/RConn3
  JOINT_D (PHI)/RConn1 -- ROD_3_BD/LConn2
  JOINT_C (THETA)/LConn1 -- GROUND_C/RConn1
  meas_JA/LConn1 -- JOINT_A (DELTA)/RConn2
  meas_JD/LConn1 -- JOINT_D (PHI)/RConn2
  ROD_3_BD/LConn1 -- JOINT_B/RConn1
  meas_JA/LConn2 -- JOINT_A (DELTA)/RConn3
  GROUND_D/RConn1 -- JOINT_D (PHI)/LConn1
  JOINT_C (THETA)/RConn2 -- meas_JC/LConn1
  ROD_2_AB/LConn1 -- meas node_A/LConn1 -- JOINT_A (DELTA)/RConn1
  ROD_1_CA/LConn2 -- JOINT_C (THETA)/RConn1
  Simulink-PS Converter/RConn1 -- JOINT_C (THETA)/LConn2
  meas_JC/LConn2 -- JOINT_C (THETA)/RConn3
  ROD_1_CA/LConn1 -- JOINT_A (DELTA)/LConn1
  JOINT_B/LConn1 -- meas node_A1/LConn1 -- ROD_2_AB/LConn2

== system bh_4bar_model_DYN/Hand_model/EYES_HAND ==
  theta_rad : Inport
  phi_rad : Inport  Port=2
  alpha_rad : Inport  Port=3
  HAND Theta_Phi_Alpha : Scope  NumInputPorts=4
  Radians to Degrees : simulink_extras/Transformations/Radians to Degrees
  Radians to Degrees1 : simulink_extras/Transformations/Radians to Degrees
  Radians to Degrees2 : simulink_extras/Transformations/Radians to Degrees
  wrap_pm_180_DEG_angle : bh_4bar_SL_LIB/4bar_basics/wrap_pm_180_DEG_angle  SystemSampleTime=-1  VariantActivationTime=update diagram  Latency=0  AutoFrameSizeCalculation=off
  wrap_pm_180_DEG_angle1 : bh_4bar_SL_LIB/4bar_basics/wrap_pm_180_DEG_angle  SystemSampleTime=-1  VariantActivationTime=update diagram  Latency=0  AutoFrameSizeCalculation=off
  wrap_pm_180_DEG_angle2 : bh_4bar_SL_LIB/4bar_basics/wrap_pm_180_DEG_angle  SystemSampleTime=-1  VariantActivationTime=update diagram  Latency=0  AutoFrameSizeCalculation=off
  THETA_deg : Outport  VectorParamsAs1DForOutWhenUnconnected=off
  PHI_deg : Outport  Port=2  VectorParamsAs1DForOutWhenUnconnected=off
  ALPHA_deg : Outport  Port=3  VectorParamsAs1DForOutWhenUnconnected=off
  wires:
  theta_rad/1 -> Radians to Degrees/1
  alpha_rad/1 -> Radians to Degrees2/1
  phi_rad/1 -> Radians to Degrees1/1
  Radians to Degrees/1 -> wrap_pm_180_DEG_angle/1, HAND Theta_Phi_Alpha/1
  Radians to Degrees1/1 -> wrap_pm_180_DEG_angle1/1
  Radians to Degrees2/1 -> wrap_pm_180_DEG_angle2/1
  wrap_pm_180_DEG_angle/1 -> HAND Theta_Phi_Alpha/2, THETA_deg/1  "THETA_deg"
  wrap_pm_180_DEG_angle1/1 -> HAND Theta_Phi_Alpha/3, PHI_deg/1  "PHI_deg"
  wrap_pm_180_DEG_angle2/1 -> HAND Theta_Phi_Alpha/4, ALPHA_deg/1  "ALPHA_deg"

== system bh_4bar_model_DYN/Hand_model/Subsystem ==
  THETA_deg : Inport
  PHI_deg : Inport  Port=2
  ALPHA_deg : Inport  Port=3
  Bus Creator : BusCreator  Inputs=3
  ANG_BUS : Outport  VectorParamsAs1DForOutWhenUnconnected=off
  wires:
  ALPHA_deg/1 -> Bus Creator/3  "ALPHA_deg"
  PHI_deg/1 -> Bus Creator/2  "PHI_deg"
  THETA_deg/1 -> Bus Creator/1  "THETA_deg"
  Bus Creator/1 -> ANG_BUS/1

== system bh_4bar_model_DYN/Hand_model/Subsystem1 ==
  theta : Inport
  theta_dot : Inport  Port=2
  Constant1 : Constant  Value=alpha_rad
  Constant12 : Constant  Value=phi_rad
  Constant13 : Constant  Value=L1
  Constant14 : Constant  Value=L2
  Constant16 : Constant  Value=L3
  Integrator : Integrator  InitialConditionSource=external
  Integrator1 : Integrator  InitialConditionSource=external
  SYS_calc_alpha_phi_DOT : bh_4bar_SL_LIB/4bar_basics/SYS_calc_alpha_phi_DOT  SystemSampleTime=-1  VariantActivationTime=update diagram  Latency=0  AutoFrameSizeCalculation=off
  alpha : Outport  VectorParamsAs1DForOutWhenUnconnected=off
  phi : Outport  Port=2  VectorParamsAs1DForOutWhenUnconnected=off
  wires:
  Constant16/1 -> SYS_calc_alpha_phi_DOT/3
  Constant14/1 -> SYS_calc_alpha_phi_DOT/2
  Constant13/1 -> SYS_calc_alpha_phi_DOT/1
  theta/1 -> SYS_calc_alpha_phi_DOT/4
  Integrator/1 -> SYS_calc_alpha_phi_DOT/5, alpha/1
  Integrator1/1 -> SYS_calc_alpha_phi_DOT/6, phi/1
  theta_dot/1 -> SYS_calc_alpha_phi_DOT/7
  Constant12/1 -> Integrator1/2
  Constant1/1 -> Integrator/2
  SYS_calc_alpha_phi_DOT/1 -> Integrator/1
  SYS_calc_alpha_phi_DOT/2 -> Integrator1/1

== system bh_4bar_model_DYN/Hand_model_LAG_CONSTRAINTS_A_b/CHECK_CONSTRAINTS ==
  L1 : Inport
  L2 : Inport  Port=2
  L3 : Inport  Port=3
  L4 : Inport  Port=4
  THETA : Inport  Port=5
  ALPHA : Inport  Port=6
  PHI : Inport  Port=7
  MATLAB Function : MATLAB Function  TreatAsAtomicUnit=on
  Scope : Scope  NumInputPorts=2
  wires:
  L4/1 -> MATLAB Function/4(L_4)
  L3/1 -> MATLAB Function/3(L_3)
  L2/1 -> MATLAB Function/2(L_2)
  L1/1 -> MATLAB Function/1(L_1)
  THETA/1 -> MATLAB Function/5(THETA)
  ALPHA/1 -> MATLAB Function/6(ALPHA)
  PHI/1 -> MATLAB Function/7(PHI)
  MATLAB Function/1(EQ_X) -> Scope/1  "EQ_X"
  MATLAB Function/2(EQ_Y) -> Scope/2  "EQ_Y"

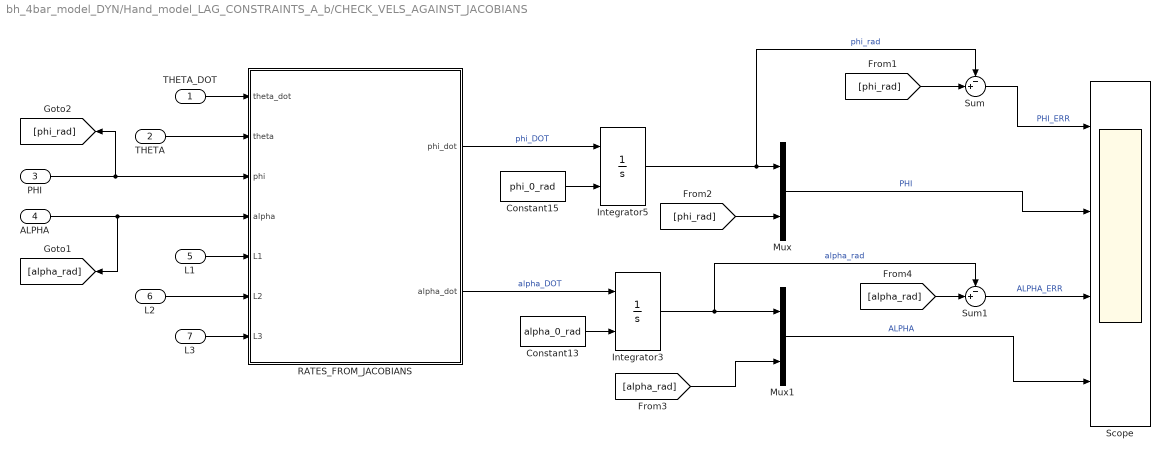
== system bh_4bar_model_DYN/Hand_model_LAG_CONSTRAINTS_A_b/CHECK_VELS_AGAINST_JACOBIANS ==
  THETA_DOT : Inport
  THETA : Inport  Port=2
  PHI : Inport  Port=3
  ALPHA : Inport  Port=4
  L1 : Inport  Port=5
  L2 : Inport  Port=6
  L3 : Inport  Port=7
  Constant13 : Constant  Value=alpha_0_rad
  Constant15 : Constant  Value=phi_0_rad
  Integrator3 : Integrator  InitialConditionSource=external  WrapState=on
  Integrator5 : Integrator  InitialConditionSource=external  WrapState=on
  Mux : Mux  Inputs=2
  Mux1 : Mux  Inputs=2
  RATES_FROM_JACOBIANS : MATLAB Function  TreatAsAtomicUnit=on
  Scope : Scope  NumInputPorts=4
  Sum : Sum  Inputs=-+|
  Sum1 : Sum  Inputs=-+|
  wires:
  L3/1 -> RATES_FROM_JACOBIANS/7(L3)
  L2/1 -> RATES_FROM_JACOBIANS/6(L2)
  L1/1 -> RATES_FROM_JACOBIANS/5(L1)
  THETA_DOT/1 -> RATES_FROM_JACOBIANS/1(theta_dot)
  THETA/1 -> RATES_FROM_JACOBIANS/2(theta)
  PHI/1 -> [phi_rad], RATES_FROM_JACOBIANS/3(phi)
  ALPHA/1 -> [alpha_rad], RATES_FROM_JACOBIANS/4(alpha)
  Constant13/1 -> Integrator3/2
  RATES_FROM_JACOBIANS/2(alpha_dot) -> Integrator3/1  "alpha_DOT"
  RATES_FROM_JACOBIANS/1(phi_dot) -> Integrator5/1  "phi_DOT"
  Integrator5/1 -> Sum/1, Mux/1  "phi_rad"
  Constant15/1 -> Integrator5/2
  [phi_rad] -> Mux/2
  Integrator3/1 -> Sum1/1, Mux1/1  "alpha_rad"
  [alpha_rad] -> Mux1/2
  [phi_rad] -> Sum/2
  Mux/1 -> Scope/2  "PHI"
  Sum/1 -> Scope/1  "PHI_ERR"
  Sum1/1 -> Scope/3  "ALPHA_ERR"
  [alpha_rad] -> Sum1/2
  Mux1/1 -> Scope/4  "ALPHA"

== system bh_4bar_model_DYN/Hand_model_LAG_CONSTRAINTS_A_b/EYES_HAND ==
  theta_rad : Inport
  phi_rad : Inport  Port=2
  alpha_rad : Inport  Port=3
  HAND Theta_Phi_Alpha : Scope  NumInputPorts=4
  Radians to Degrees : simulink_extras/Transformations/Radians to Degrees
  Radians to Degrees1 : simulink_extras/Transformations/Radians to Degrees
  Radians to Degrees2 : simulink_extras/Transformations/Radians to Degrees
  wrap_pm_180_DEG_angle : bh_4bar_SL_LIB/4bar_basics/wrap_pm_180_DEG_angle  SystemSampleTime=-1  VariantActivationTime=update diagram  Latency=0  AutoFrameSizeCalculation=off
  wrap_pm_180_DEG_angle1 : bh_4bar_SL_LIB/4bar_basics/wrap_pm_180_DEG_angle  SystemSampleTime=-1  VariantActivationTime=update diagram  Latency=0  AutoFrameSizeCalculation=off
  wrap_pm_180_DEG_angle2 : bh_4bar_SL_LIB/4bar_basics/wrap_pm_180_DEG_angle  SystemSampleTime=-1  VariantActivationTime=update diagram  Latency=0  AutoFrameSizeCalculation=off
  THETA_deg : Outport  VectorParamsAs1DForOutWhenUnconnected=off
  PHI_deg : Outport  Port=2  VectorParamsAs1DForOutWhenUnconnected=off
  ALPHA_deg : Outport  Port=3  VectorParamsAs1DForOutWhenUnconnected=off
  wires:
  theta_rad/1 -> Radians to Degrees/1
  alpha_rad/1 -> Radians to Degrees2/1
  phi_rad/1 -> Radians to Degrees1/1
  Radians to Degrees/1 -> wrap_pm_180_DEG_angle/1, HAND Theta_Phi_Alpha/1
  Radians to Degrees1/1 -> wrap_pm_180_DEG_angle1/1
  Radians to Degrees2/1 -> wrap_pm_180_DEG_angle2/1
  wrap_pm_180_DEG_angle/1 -> HAND Theta_Phi_Alpha/2, THETA_deg/1  "THETA_deg"
  wrap_pm_180_DEG_angle1/1 -> HAND Theta_Phi_Alpha/3, PHI_deg/1  "PHI_deg"
  wrap_pm_180_DEG_angle2/1 -> HAND Theta_Phi_Alpha/4, ALPHA_deg/1  "ALPHA_deg"

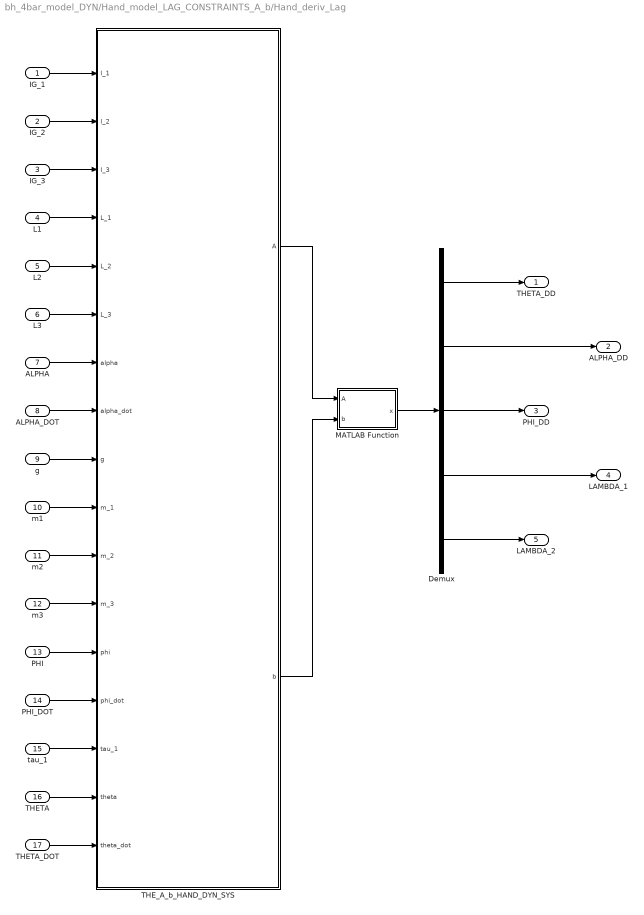
== system bh_4bar_model_DYN/Hand_model_LAG_CONSTRAINTS_A_b/Hand_deriv_Lag ==
  IG_1 : Inport
  IG_2 : Inport  Port=2
  IG_3 : Inport  Port=3
  L1 : Inport  Port=4
  L2 : Inport  Port=5
  L3 : Inport  Port=6
  ALPHA : Inport  Port=7
  ALPHA_DOT : Inport  Port=8
  g : Inport  Port=9
  m1 : Inport  Port=10
  m2 : Inport  Port=11
  m3 : Inport  Port=12
  PHI : Inport  Port=13
  PHI_DOT : Inport  Port=14
  tau_1 : Inport  Port=15
  THETA : Inport  Port=16
  THETA_DOT : Inport  Port=17
  Demux : Demux  Outputs=5
  MATLAB Function : MATLAB Function  TreatAsAtomicUnit=on
  THE_A_b_HAND_DYN_SYS : MATLAB Function  TreatAsAtomicUnit=on
  THETA_DD : Outport
  ALPHA_DD : Outport  Port=2
  PHI_DD : Outport  Port=3
  LAMBDA_1 : Outport  Port=4
  LAMBDA_2 : Outport  Port=5
  wires:
  L2/1 -> THE_A_b_HAND_DYN_SYS/5(L_2)
  IG_3/1 -> THE_A_b_HAND_DYN_SYS/3(I_3)
  L1/1 -> THE_A_b_HAND_DYN_SYS/4(L_1)
  L3/1 -> THE_A_b_HAND_DYN_SYS/6(L_3)
  ALPHA/1 -> THE_A_b_HAND_DYN_SYS/7(alpha)
  IG_2/1 -> THE_A_b_HAND_DYN_SYS/2(I_2)
  IG_1/1 -> THE_A_b_HAND_DYN_SYS/1(I_1)
  m2/1 -> THE_A_b_HAND_DYN_SYS/11(m_2)
  ALPHA_DOT/1 -> THE_A_b_HAND_DYN_SYS/8(alpha_dot)
  m1/1 -> THE_A_b_HAND_DYN_SYS/10(m_1)
  g/1 -> THE_A_b_HAND_DYN_SYS/9(g)
  tau_1/1 -> THE_A_b_HAND_DYN_SYS/15(tau_1)
  m3/1 -> THE_A_b_HAND_DYN_SYS/12(m_3)
  PHI_DOT/1 -> THE_A_b_HAND_DYN_SYS/14(phi_dot)
  PHI/1 -> THE_A_b_HAND_DYN_SYS/13(phi)
  THETA_DOT/1 -> THE_A_b_HAND_DYN_SYS/17(theta_dot)
  THETA/1 -> THE_A_b_HAND_DYN_SYS/16(theta)
  THE_A_b_HAND_DYN_SYS/1(A) -> MATLAB Function/1(A)
  THE_A_b_HAND_DYN_SYS/2(b) -> MATLAB Function/2(b)
  MATLAB Function/1(x) -> Demux/1
  Demux/1 -> THETA_DD/1
  Demux/2 -> ALPHA_DD/1
  Demux/3 -> PHI_DD/1
  Demux/4 -> LAMBDA_1/1
  Demux/5 -> LAMBDA_2/1

== system bh_4bar_model_DYN/Hand_model_LAG_CONSTRAINTS_A_b/Subsystem ==
  THETA_deg : Inport
  PHI_deg : Inport  Port=2
  ALPHA_deg : Inport  Port=3
  Bus Creator : BusCreator  Inputs=3
  ANG_BUS : Outport  VectorParamsAs1DForOutWhenUnconnected=off
  wires:
  ALPHA_deg/1 -> Bus Creator/3  "ALPHA_deg"
  PHI_deg/1 -> Bus Creator/2  "PHI_deg"
  THETA_deg/1 -> Bus Creator/1  "THETA_deg"
  Bus Creator/1 -> ANG_BUS/1

== system bh_4bar_model_DYN/Hand_model_LAG_CONSTRAINTS_invA/CHECK_CONSTRAINTS ==
  L1 : Inport
  L2 : Inport  Port=2
  L3 : Inport  Port=3
  L4 : Inport  Port=4
  THETA : Inport  Port=5
  ALPHA : Inport  Port=6
  PHI : Inport  Port=7
  MATLAB Function : MATLAB Function  TreatAsAtomicUnit=on
  Scope : Scope  NumInputPorts=2
  wires:
  L4/1 -> MATLAB Function/4(L_4)
  L3/1 -> MATLAB Function/3(L_3)
  L2/1 -> MATLAB Function/2(L_2)
  L1/1 -> MATLAB Function/1(L_1)
  THETA/1 -> MATLAB Function/5(THETA)
  ALPHA/1 -> MATLAB Function/6(ALPHA)
  PHI/1 -> MATLAB Function/7(PHI)
  MATLAB Function/1(EQ_X) -> Scope/1  "EQ_X"
  MATLAB Function/2(EQ_Y) -> Scope/2  "EQ_Y"

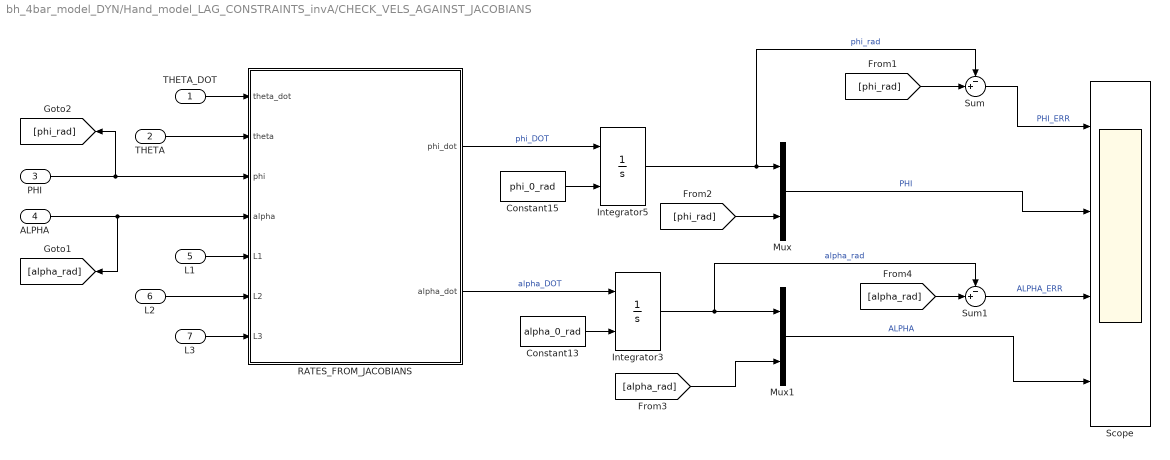
== system bh_4bar_model_DYN/Hand_model_LAG_CONSTRAINTS_invA/CHECK_VELS_AGAINST_JACOBIANS ==
  THETA_DOT : Inport
  THETA : Inport  Port=2
  PHI : Inport  Port=3
  ALPHA : Inport  Port=4
  L1 : Inport  Port=5
  L2 : Inport  Port=6
  L3 : Inport  Port=7
  Constant13 : Constant  Value=alpha_0_rad
  Constant15 : Constant  Value=phi_0_rad
  Integrator3 : Integrator  InitialConditionSource=external  WrapState=on
  Integrator5 : Integrator  InitialConditionSource=external  WrapState=on
  Mux : Mux  Inputs=2
  Mux1 : Mux  Inputs=2
  RATES_FROM_JACOBIANS : MATLAB Function  TreatAsAtomicUnit=on
  Scope : Scope  NumInputPorts=4
  Sum : Sum  Inputs=-+|
  Sum1 : Sum  Inputs=-+|
  wires:
  L3/1 -> RATES_FROM_JACOBIANS/7(L3)
  L2/1 -> RATES_FROM_JACOBIANS/6(L2)
  L1/1 -> RATES_FROM_JACOBIANS/5(L1)
  THETA_DOT/1 -> RATES_FROM_JACOBIANS/1(theta_dot)
  THETA/1 -> RATES_FROM_JACOBIANS/2(theta)
  PHI/1 -> [phi_rad], RATES_FROM_JACOBIANS/3(phi)
  ALPHA/1 -> [alpha_rad], RATES_FROM_JACOBIANS/4(alpha)
  Constant13/1 -> Integrator3/2
  RATES_FROM_JACOBIANS/2(alpha_dot) -> Integrator3/1  "alpha_DOT"
  RATES_FROM_JACOBIANS/1(phi_dot) -> Integrator5/1  "phi_DOT"
  Integrator5/1 -> Sum/1, Mux/1  "phi_rad"
  Constant15/1 -> Integrator5/2
  [phi_rad] -> Mux/2
  Integrator3/1 -> Sum1/1, Mux1/1  "alpha_rad"
  [alpha_rad] -> Mux1/2
  [phi_rad] -> Sum/2
  Mux/1 -> Scope/2  "PHI"
  Sum/1 -> Scope/1  "PHI_ERR"
  Sum1/1 -> Scope/3  "ALPHA_ERR"
  [alpha_rad] -> Sum1/2
  Mux1/1 -> Scope/4  "ALPHA"

== system bh_4bar_model_DYN/Hand_model_LAG_CONSTRAINTS_invA/EYES_HAND ==
  theta_rad : Inport
  phi_rad : Inport  Port=2
  alpha_rad : Inport  Port=3
  HAND Theta_Phi_Alpha : Scope  NumInputPorts=4
  Radians to Degrees : simulink_extras/Transformations/Radians to Degrees
  Radians to Degrees1 : simulink_extras/Transformations/Radians to Degrees
  Radians to Degrees2 : simulink_extras/Transformations/Radians to Degrees
  wrap_pm_180_DEG_angle : bh_4bar_SL_LIB/4bar_basics/wrap_pm_180_DEG_angle  SystemSampleTime=-1  Latency=0  AutoFrameSizeCalculation=off
  wrap_pm_180_DEG_angle1 : bh_4bar_SL_LIB/4bar_basics/wrap_pm_180_DEG_angle  SystemSampleTime=-1  Latency=0  AutoFrameSizeCalculation=off
  wrap_pm_180_DEG_angle2 : bh_4bar_SL_LIB/4bar_basics/wrap_pm_180_DEG_angle  SystemSampleTime=-1  Latency=0  AutoFrameSizeCalculation=off
  THETA_deg : Outport  VectorParamsAs1DForOutWhenUnconnected=off
  PHI_deg : Outport  Port=2  VectorParamsAs1DForOutWhenUnconnected=off
  ALPHA_deg : Outport  Port=3  VectorParamsAs1DForOutWhenUnconnected=off
  wires:
  theta_rad/1 -> Radians to Degrees/1
  alpha_rad/1 -> Radians to Degrees2/1
  phi_rad/1 -> Radians to Degrees1/1
  Radians to Degrees/1 -> wrap_pm_180_DEG_angle/1, HAND Theta_Phi_Alpha/1
  Radians to Degrees1/1 -> wrap_pm_180_DEG_angle1/1
  Radians to Degrees2/1 -> wrap_pm_180_DEG_angle2/1
  wrap_pm_180_DEG_angle/1 -> HAND Theta_Phi_Alpha/2, THETA_deg/1  "THETA_deg"
  wrap_pm_180_DEG_angle1/1 -> HAND Theta_Phi_Alpha/3, PHI_deg/1  "PHI_deg"
  wrap_pm_180_DEG_angle2/1 -> HAND Theta_Phi_Alpha/4, ALPHA_deg/1  "ALPHA_deg"

== system bh_4bar_model_DYN/Hand_model_LAG_CONSTRAINTS_invA/Subsystem ==
  THETA_deg : Inport
  PHI_deg : Inport  Port=2
  ALPHA_deg : Inport  Port=3
  Bus Creator : BusCreator  Inputs=3
  ANG_BUS : Outport  VectorParamsAs1DForOutWhenUnconnected=off
  wires:
  ALPHA_deg/1 -> Bus Creator/3  "ALPHA_deg"
  PHI_deg/1 -> Bus Creator/2  "PHI_deg"
  THETA_deg/1 -> Bus Creator/1  "THETA_deg"
  Bus Creator/1 -> ANG_BUS/1

== system bh_4bar_model_DYN/Simscape_model/CHECK_CONSTRAINTS ==
  L1 : Inport
  L2 : Inport  Port=2
  L3 : Inport  Port=3
  L4 : Inport  Port=4
  THETA : Inport  Port=5
  ALPHA : Inport  Port=6
  PHI : Inport  Port=7
  MATLAB Function : MATLAB Function  TreatAsAtomicUnit=on
  Scope : Scope  NumInputPorts=2
  wires:
  L4/1 -> MATLAB Function/4(L_4)
  L3/1 -> MATLAB Function/3(L_3)
  L2/1 -> MATLAB Function/2(L_2)
  L1/1 -> MATLAB Function/1(L_1)
  THETA/1 -> MATLAB Function/5(THETA)
  ALPHA/1 -> MATLAB Function/6(ALPHA)
  PHI/1 -> MATLAB Function/7(PHI)
  MATLAB Function/1(EQ_X) -> Scope/1  "EQ_X"
  MATLAB Function/2(EQ_Y) -> Scope/2  "EQ_Y"
